simulink model "P7_struct_unc_model"  (R2024b)
settings: Solver=VariableStepAuto  StartTime=0.0  StopTime=10.0  RelTol=1e-3
values from neighbouring files (symbols this model uses):
  Kn = (Ku(1)+Ku(2))/2    [P7.m]
  p1n = (p1u(1)+p1u(2))/2    [P7.m]
  p2n = (p2u(1)+p2u(2))/2    [P7.m]
  Wk = (Ku(2)-Kn)/Kn    [P7.m]
  Wp1 = (p1u(2)-p1n)/p1n    [P7.m]
  Wp2 = (p2u(2)-p2n)/p2n    [P7.m]
settings Model: Creator=lucap  LastModifiedBy=lucap

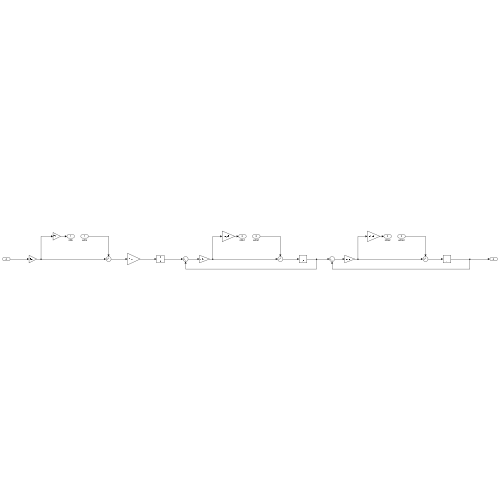
[thumbnail: Simulink's stored preview of the top-level diagram]
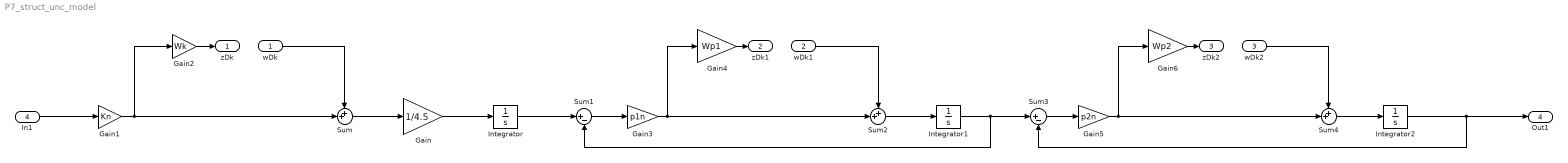
== system P7_struct_unc_model ==
  wDk : Inport
  wDk1 : Inport  Port=2
  wDk2 : Inport  Port=3
  In1 : Inport  Port=4
  Gain : Gain  Gain=1/4.5
  Gain1 : Gain  Gain=Kn
  Gain2 : Gain  Gain=Wk
  Gain3 : Gain  Gain=p1n
  Gain4 : Gain  Gain=Wp1
  Gain5 : Gain  Gain=p2n
  Gain6 : Gain  Gain=Wp2
  Integrator : Integrator
  Integrator1 : Integrator
  Integrator2 : Integrator
  Sum : Sum  Inputs=++|
  Sum1 : Sum  Inputs=|+-
  Sum2 : Sum  Inputs=++|
  Sum3 : Sum  Inputs=|+-
  Sum4 : Sum  Inputs=++|
  zDk : Outport
  zDk1 : Outport  Port=2
  zDk2 : Outport  Port=3
  Out1 : Outport  Port=4
  wires:
  Gain1/1 -> Sum/2, Gain2/1
  Gain2/1 -> zDk/1
  wDk/1 -> Sum/1
  Sum/1 -> Gain/1
  Gain/1 -> Integrator/1
  Integrator/1 -> Sum1/1
  Gain4/1 -> zDk1/1
  Gain3/1 -> Sum2/2, Gain4/1
  wDk1/1 -> Sum2/1
  Sum1/1 -> Gain3/1
  Sum2/1 -> Integrator1/1
  Integrator1/1 -> Sum1/2, Sum3/1
  Gain6/1 -> zDk2/1
  Gain5/1 -> Sum4/2, Gain6/1
  wDk2/1 -> Sum4/1
  Sum3/1 -> Gain5/1
  Sum4/1 -> Integrator2/1
  In1/1 -> Gain1/1
  Integrator2/1 -> Sum3/2, Out1/1
